simulink model "dreg"  (R2024b)
settings: Solver=FixedStepDiscrete  StartTime=tspan(1)  StopTime=tspan(2)  FixedStep=T_vz  RelTol=1e-3
values from neighbouring files (symbols this model uses):
  desr = [35 40]    [motor.m]
  desr_val = 0.01    [motor.m]
  dtf = c2d(tfun, T_vz, 'tustin')    [motor.m]
  PSDReg = PSD(GhReg, Ts_reg)    [motor.m]
  step_t = 5    [motor.m]
settings Model: Creator=markminerov  LastModifiedBy=markminerov
settings DebuggingCC: AlgebraicLoopMsg=none

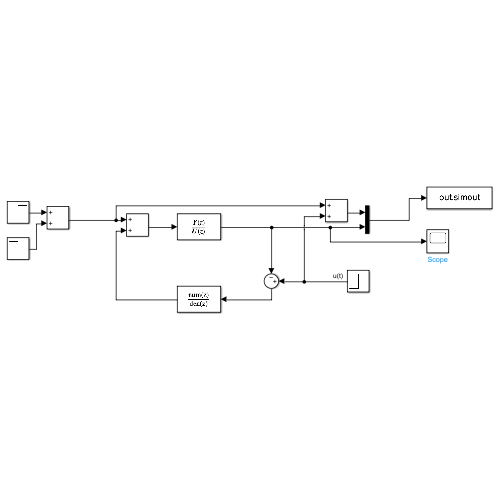
[thumbnail: Simulink's stored preview of the top-level diagram]
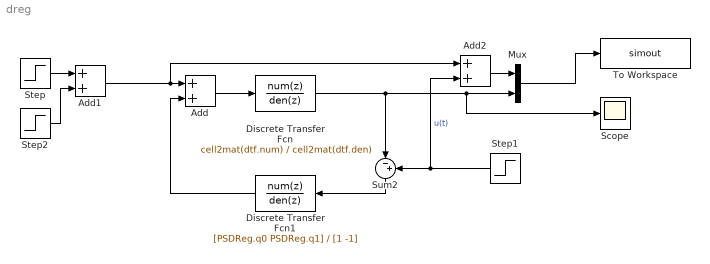
== system dreg ==
  Add : Sum
  Add1 : Sum
  Add2 : Sum
  Discrete Transfer Fcn : DiscreteTransferFcn  Numerator=cell2mat(dtf.num)  Denominator=cell2mat(dtf.den)
  Discrete Transfer Fcn1 : DiscreteTransferFcn  Numerator=[PSDReg.q0 PSDReg.q1]  Denominator=[1 -1]
  Mux : Mux  Inputs=2
  Scope : Scope
  Step : Step  Time=desr(2)  After=desr_val  SampleTime=0
  Step1 : Step  Time=step_t  After=u  SampleTime=0
  Step2 : Step  Time=desr(1)  After=-desr_val  SampleTime=0
  Sum2 : Sum  Inputs=|-+
  To Workspace : ToWorkspace  VariableName=simout  SaveFormat=Timeseries  SampleTime=-1
  wires:
  Discrete Transfer Fcn1/1 -> Add/2
  Discrete Transfer Fcn/1 -> Scope/1, Mux/2, Sum2/1
  Sum2/1 -> Discrete Transfer Fcn1/1
  Step1/1 -> Add2/2, Sum2/2  "u(t)"
  Add/1 -> Discrete Transfer Fcn/1
  Step/1 -> Add1/1
  Step2/1 -> Add1/2
  Add1/1 -> Add2/1, Add/1
  Add2/1 -> Mux/1
  Mux/1 -> To Workspace/1
